simulink model "InverterInputs"  (R2024b)
settings: Solver=FixedStepAuto  StartTime=0.0  StopTime=10.0  RelTol=1e-3  EnableMultiTasking=on
settings Model: DataDictionary=Master_Dictionary.sldd  EnableAccessToBaseWorkspace=off  Creator=torni  LastModifiedBy=Will
settings OptimizationCC: DefaultParameterBehavior=Inlined  EnhancedBackFolding=on  PassReuseOutputArgsAs=Individual arguments  ZeroExternalMemoryAtStartup=off  ZeroInternalMemoryAtStartup=off  MaxStackSize=8192  OptimizeBlockOrder=speed  DifferentSizesBufferReuse=on  OptimizationCustomize=off  EfficientTunableParamExpr=on
settings DebuggingCC: ParameterTunabilityLossMsg=error
settings HardwareCC: ProdBitPerPointer=32  ProdBitPerSizeT=32  ProdBitPerPtrDiffT=32  ProdLargestAtomicInteger=Long  ProdLargestAtomicFloat=Double  ProdWordSize=32  ProdLongLongMode=on  ProdHWDeviceType=ARM Compatible->ARM Cortex-M
settings SFSimCC: MATLABDynamicMemAlloc=off
settings RTWCC: Description=Embedded Coder  SystemTargetFile=ert.tlc  HardwareBoard=STM32H7xx Based (Single-core)  TemplateMakefile=ert_default_tmf  Toolchain=GNU Tools for ARM Embedded Processors
settings CodeAppCC: ForceParamTrailComments=on  IgnoreCustomStorageClasses=off  OperatorAnnotations=on  SimulinkDataObjDesc=on  SFDataObjDesc=on  InsertBlockDesc=on
settings ERTTargetCC: TargetLangStandard=C99 (ISO)  CodeReplacementLibrary=ARM Cortex-M  ExtModeTransport=3  ExtModeStaticAlloc=on  ExtModeStaticAllocSize=2048  ExtModeMexFile=ext_xcp  ExtModeIntrfLevel=Level2 - Open

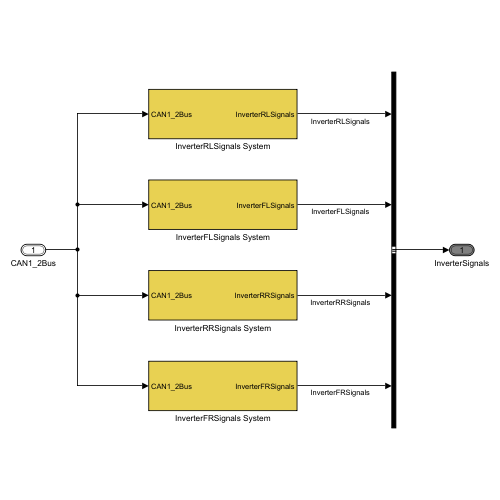
[thumbnail: Simulink's stored preview of the top-level diagram]
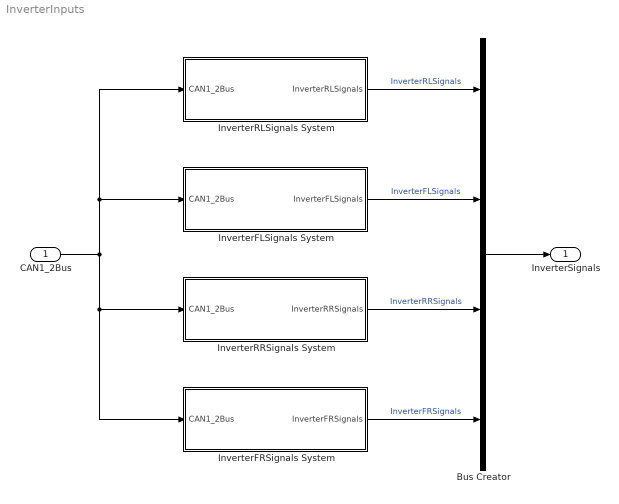
== system InverterInputs ==
  CAN1_2Bus : Inport  OutDataTypeStr=Bus: CAN1_2Bus
  Bus Creator : BusCreator  Inputs=4  OutDataTypeStr=Bus: InverterSignals
  InverterFLSignals System : Subsystem
  InverterFRSignals System : Subsystem
  InverterRLSignals System : Subsystem
  InverterRRSignals System : Subsystem
  InverterSignals : Outport  OutDataTypeStr=Bus: InverterSignals  VectorParamsAs1DForOutWhenUnconnected=off
  wires:
  InverterRLSignals System/1(InverterRLSignals) -> Bus Creator/1  "InverterRLSignals"
  InverterRRSignals System/1(InverterRRSignals) -> Bus Creator/3  "InverterRRSignals"
  InverterFRSignals System/1(InverterFRSignals) -> Bus Creator/4  "InverterFRSignals"
  InverterFLSignals System/1(InverterFLSignals) -> Bus Creator/2  "InverterFLSignals"
  Bus Creator/1 -> InverterSignals/1
  CAN1_2Bus/1 -> InverterFLSignals System/1(CAN1_2Bus), InverterRLSignals System/1(CAN1_2Bus), InverterRRSignals System/1(CAN1_2Bus), InverterFRSignals System/1(CAN1_2Bus)

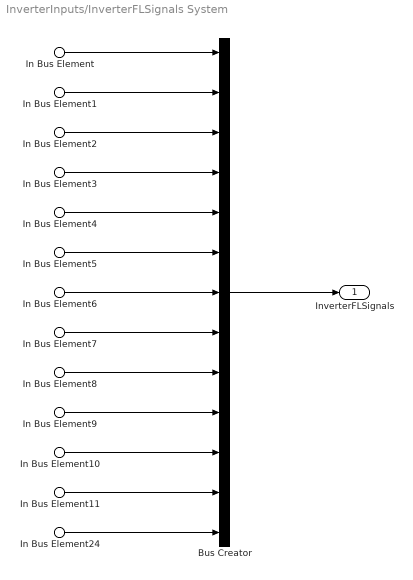
== system InverterInputs/InverterFLSignals System ==
  In Bus Element : Inport  PortName=CAN1_2Bus  Element=InverterFL.nMotorFL
  In Bus Element1 : Inport  PortName=CAN1_2Bus  Element=InverterFL.BInvDCOnFLIn
  In Bus Element2 : Inport  PortName=CAN1_2Bus  Element=InverterFL.BInvErrorFL
  In Bus Element3 : Inport  PortName=CAN1_2Bus  Element=InverterFL.BInvOnFLIn
  In Bus Element4 : Inport  PortName=CAN1_2Bus  Element=InverterFL.BInvQuitDcOnFL
  In Bus Element5 : Inport  PortName=CAN1_2Bus  Element=InverterFL.BQuitInvOnFL
  In Bus Element6 : Inport  PortName=CAN1_2Bus  Element=InverterFL.BInvSysReadyFL
  In Bus Element7 : Inport  PortName=CAN1_2Bus  Element=InverterFL.BInvWarnFL
  In Bus Element8 : Inport  PortName=CAN1_2Bus  Element=InverterFL.MMotorMeasuredFL
  In Bus Element9 : Inport  PortName=CAN1_2Bus  Element=InverterFL.NInvDTCFL
  In Bus Element10 : Inport  PortName=CAN1_2Bus  Element=InverterFL.TMotorFL
  In Bus Element11 : Inport  PortName=CAN1_2Bus  Element=InverterFL.VDCInvFL
  In Bus Element24 : Inport  PortName=CAN1_2Bus  Element=InverterFL.TInvFL
  Bus Creator : BusCreator  Inputs=13  OutDataTypeStr=Bus: InverterFLSignals
  InverterFLSignals : Outport  OutDataTypeStr=Bus: InverterFLSignals  VectorParamsAs1DForOutWhenUnconnected=off
  wires:
  Bus Creator/1 -> InverterFLSignals/1
  In Bus Element/1 -> Bus Creator/1
  In Bus Element10/1 -> Bus Creator/11
  In Bus Element11/1 -> Bus Creator/12
  In Bus Element24/1 -> Bus Creator/13
  In Bus Element8/1 -> Bus Creator/9
  In Bus Element7/1 -> Bus Creator/8
  In Bus Element6/1 -> Bus Creator/7
  In Bus Element5/1 -> Bus Creator/6
  In Bus Element4/1 -> Bus Creator/5
  In Bus Element3/1 -> Bus Creator/4
  In Bus Element2/1 -> Bus Creator/3
  In Bus Element1/1 -> Bus Creator/2
  In Bus Element9/1 -> Bus Creator/10

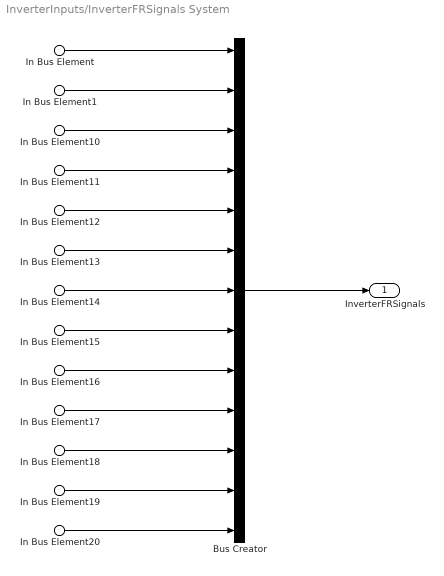
== system InverterInputs/InverterFRSignals System ==
  In Bus Element : Inport  PortName=CAN1_2Bus  Element=InverterFR.nMotorFR
  In Bus Element1 : Inport  PortName=CAN1_2Bus  Element=InverterFR.BInvDCOnFRIn
  In Bus Element10 : Inport  PortName=CAN1_2Bus  Element=InverterFR.BInvErrorFR
  In Bus Element11 : Inport  PortName=CAN1_2Bus  Element=InverterFR.BInvOnFRIn
  In Bus Element12 : Inport  PortName=CAN1_2Bus  Element=InverterFR.BInvQuitDcOnFR
  In Bus Element13 : Inport  PortName=CAN1_2Bus  Element=InverterFR.BQuitInvOnFR
  In Bus Element14 : Inport  PortName=CAN1_2Bus  Element=InverterFR.BInvSysReadyFR
  In Bus Element15 : Inport  PortName=CAN1_2Bus  Element=InverterFR.BInvWarnFR
  In Bus Element16 : Inport  PortName=CAN1_2Bus  Element=InverterFR.MMotorMeasuredFR
  In Bus Element17 : Inport  PortName=CAN1_2Bus  Element=InverterFR.NInvDTCFR
  In Bus Element18 : Inport  PortName=CAN1_2Bus  Element=InverterFR.TMotorFR
  In Bus Element19 : Inport  PortName=CAN1_2Bus  Element=InverterFR.VDCInvFR
  In Bus Element20 : Inport  PortName=CAN1_2Bus  Element=InverterFR.TInvFR
  Bus Creator : BusCreator  Inputs=13  OutDataTypeStr=Bus: InverterFRSignals
  InverterFRSignals : Outport  OutDataTypeStr=Bus: InverterFRSignals  VectorParamsAs1DForOutWhenUnconnected=off
  wires:
  Bus Creator/1 -> InverterFRSignals/1
  In Bus Element/1 -> Bus Creator/1
  In Bus Element1/1 -> Bus Creator/2
  In Bus Element11/1 -> Bus Creator/4
  In Bus Element12/1 -> Bus Creator/5
  In Bus Element13/1 -> Bus Creator/6
  In Bus Element14/1 -> Bus Creator/7
  In Bus Element15/1 -> Bus Creator/8
  In Bus Element16/1 -> Bus Creator/9
  In Bus Element17/1 -> Bus Creator/10
  In Bus Element18/1 -> Bus Creator/11
  In Bus Element19/1 -> Bus Creator/12
  In Bus Element10/1 -> Bus Creator/3
  In Bus Element20/1 -> Bus Creator/13

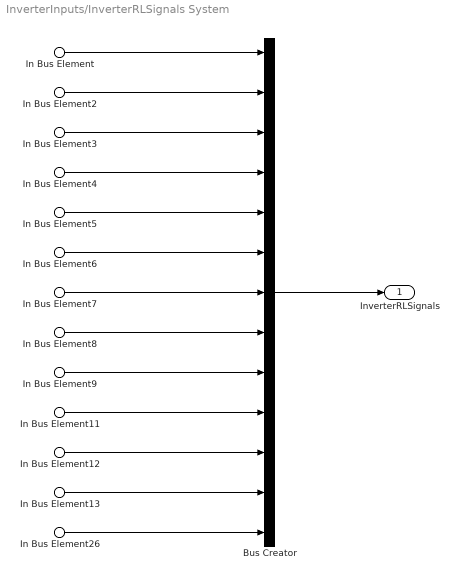
== system InverterInputs/InverterRLSignals System ==
  In Bus Element : Inport  PortName=CAN1_2Bus  Element=InverterRL.nMotorRL
  In Bus Element2 : Inport  PortName=CAN1_2Bus  Element=InverterRL.BInvDCOnRLIn
  In Bus Element3 : Inport  PortName=CAN1_2Bus  Element=InverterRL.BInvErrorRL
  In Bus Element4 : Inport  PortName=CAN1_2Bus  Element=InverterRL.BInvOnRLIn
  In Bus Element5 : Inport  PortName=CAN1_2Bus  Element=InverterRL.BInvQuitDcOnRL
  In Bus Element6 : Inport  PortName=CAN1_2Bus  Element=InverterRL.BQuitInvOnRL
  In Bus Element7 : Inport  PortName=CAN1_2Bus  Element=InverterRL.BInvSysReadyRL
  In Bus Element8 : Inport  PortName=CAN1_2Bus  Element=InverterRL.BInvWarnRL
  In Bus Element9 : Inport  PortName=CAN1_2Bus  Element=InverterRL.MMotorMeasuredRL
  In Bus Element11 : Inport  PortName=CAN1_2Bus  Element=InverterRL.NInvDTCRL
  In Bus Element12 : Inport  PortName=CAN1_2Bus  Element=InverterRL.TMotorRL
  In Bus Element13 : Inport  PortName=CAN1_2Bus  Element=InverterRL.VDCInvRL
  In Bus Element26 : Inport  PortName=CAN1_2Bus  Element=InverterRL.TInvRL
  Bus Creator : BusCreator  Inputs=13  OutDataTypeStr=Bus: InverterRLSignals
  InverterRLSignals : Outport  OutDataTypeStr=Bus: InverterRLSignals  VectorParamsAs1DForOutWhenUnconnected=off
  wires:
  Bus Creator/1 -> InverterRLSignals/1
  In Bus Element/1 -> Bus Creator/1
  In Bus Element2/1 -> Bus Creator/2
  In Bus Element3/1 -> Bus Creator/3
  In Bus Element4/1 -> Bus Creator/4
  In Bus Element5/1 -> Bus Creator/5
  In Bus Element6/1 -> Bus Creator/6
  In Bus Element7/1 -> Bus Creator/7
  In Bus Element8/1 -> Bus Creator/8
  In Bus Element9/1 -> Bus Creator/9
  In Bus Element12/1 -> Bus Creator/11
  In Bus Element13/1 -> Bus Creator/12
  In Bus Element26/1 -> Bus Creator/13
  In Bus Element11/1 -> Bus Creator/10

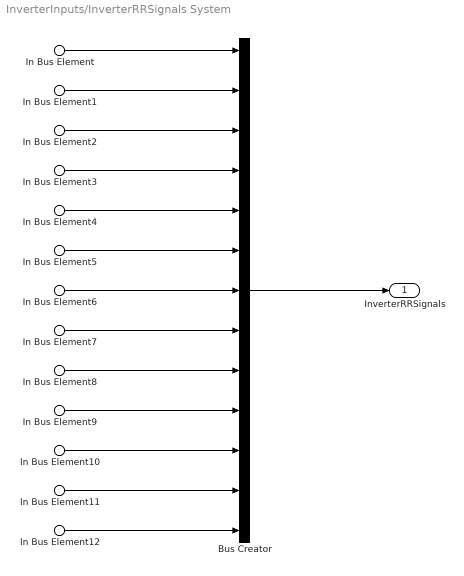
== system InverterInputs/InverterRRSignals System ==
  In Bus Element : Inport  PortName=CAN1_2Bus  Element=InverterRR.nMotorRR
  In Bus Element1 : Inport  PortName=CAN1_2Bus  Element=InverterRR.BInvDCOnRRIn
  In Bus Element2 : Inport  PortName=CAN1_2Bus  Element=InverterRR.BInvErrorRR
  In Bus Element3 : Inport  PortName=CAN1_2Bus  Element=InverterRR.BInvOnRRIn
  In Bus Element4 : Inport  PortName=CAN1_2Bus  Element=InverterRR.BInvQuitDcOnRR
  In Bus Element5 : Inport  PortName=CAN1_2Bus  Element=InverterRR.BQuitInvOnRR
  In Bus Element6 : Inport  PortName=CAN1_2Bus  Element=InverterRR.BInvSysReadyRR
  In Bus Element7 : Inport  PortName=CAN1_2Bus  Element=InverterRR.BInvWarnRR
  In Bus Element8 : Inport  PortName=CAN1_2Bus  Element=InverterRR.MMotorMeasuredRR
  In Bus Element9 : Inport  PortName=CAN1_2Bus  Element=InverterRR.NInvDTCRR
  In Bus Element10 : Inport  PortName=CAN1_2Bus  Element=InverterRR.TMotorRR
  In Bus Element11 : Inport  PortName=CAN1_2Bus  Element=InverterRR.VDCInvRR
  In Bus Element12 : Inport  PortName=CAN1_2Bus  Element=InverterRR.TInvRR
  Bus Creator : BusCreator  Inputs=13  OutDataTypeStr=Bus: InverterRRSignals
  InverterRRSignals : Outport  OutDataTypeStr=Bus: InverterRRSignals  VectorParamsAs1DForOutWhenUnconnected=off
  wires:
  Bus Creator/1 -> InverterRRSignals/1
  In Bus Element/1 -> Bus Creator/1
  In Bus Element1/1 -> Bus Creator/2
  In Bus Element2/1 -> Bus Creator/3
  In Bus Element3/1 -> Bus Creator/4
  In Bus Element4/1 -> Bus Creator/5
  In Bus Element5/1 -> Bus Creator/6
  In Bus Element6/1 -> Bus Creator/7
  In Bus Element7/1 -> Bus Creator/8
  In Bus Element8/1 -> Bus Creator/9
  In Bus Element9/1 -> Bus Creator/10
  In Bus Element10/1 -> Bus Creator/11
  In Bus Element11/1 -> Bus Creator/12
  In Bus Element12/1 -> Bus Creator/13
